simulink model "mppt"  (R2015a)
settings: Solver=ode23tb  StartTime=0.0  StopTime=1.0  RelTol=1e-3
libraries: powerlib x11, simulink x2
settings Model: Creator=Dell  LastModifiedBy=Dell

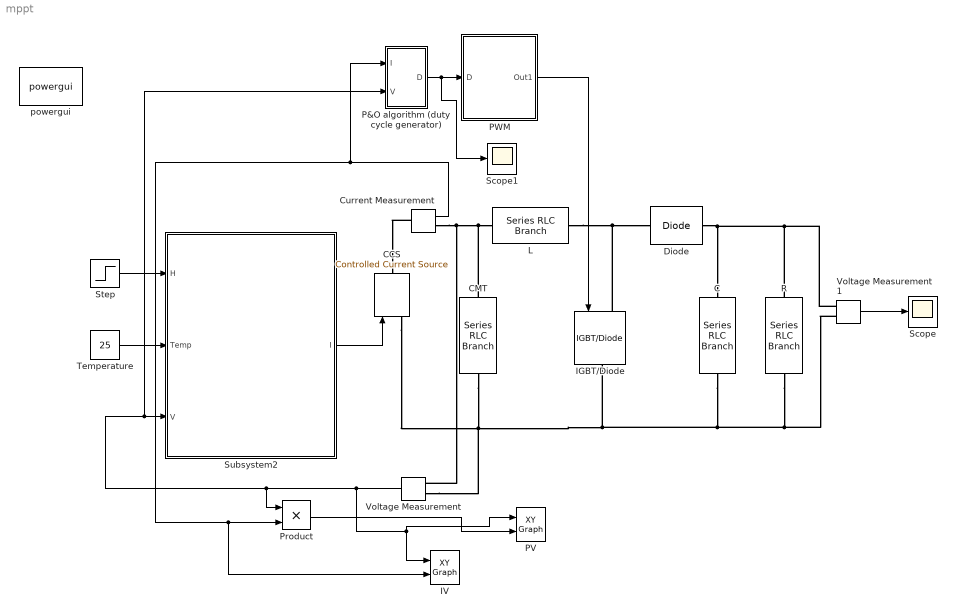
== system mppt ==
  C : powerlib/Elements/Series RLC Branch  LConnTagsString=__new0  RConnTagsString=__new0  BranchType=C  Resistance=1  Inductance=1e-3  SetiL0=off  InitialCurrent=0  Capacitance=1000e-6  Setx0=off  InitialVoltage=0  Measurements=None
  CCS : powerlib/Electrical Sources/Controlled Current Source  Initialize=on  Source_Type=AC  Amplitude=0  Phase=0  Frequency=0  Measurements=None
  CMT : powerlib/Elements/Series RLC Branch  LConnTagsString=__new0  RConnTagsString=__new0  BranchType=C  Resistance=1  Inductance=1e-3  SetiL0=off  InitialCurrent=0  Capacitance=1000e-6  Setx0=off  InitialVoltage=0  Measurements=None
  Current Measurement : powerlib/Measurements/Current Measurement  PhasorSimulation=off  OutputType=Complex  PSBequivalent=0
  Diode : powerlib/Power Electronics/Diode  Ron=0.001  Lon=0  Vf=0.8  IC=0  UseSnubber=off  Rs=500  Cs=250e-9  Measurements=off
  IGBT/Diode : powerlib/Power Electronics/IGBT//Diode  Ron=1e-3  Rs=1e5  Cs=inf  Measurements=off
  IV : simulink/Sinks/XY Graph  xmin=0  xmax=30  ymin=0  ymax=8  st=-1
  L : powerlib/Elements/Series RLC Branch  LConnTagsString=__new0  RConnTagsString=__new0  BranchType=L  Resistance=1  Inductance=4e-4  SetiL0=off  InitialCurrent=0  Capacitance=1e-6  Setx0=off  InitialVoltage=0  Measurements=None
  P&O algorithm (duty cycle generator) : Subsystem
  PV : simulink/Sinks/XY Graph  xmin=0  xmax=20  ymin=0  ymax=75  st=-1
  PWM : Subsystem
  Product : Product
  R : powerlib/Elements/Series RLC Branch  LConnTagsString=__new0  RConnTagsString=__new0  BranchType=R  Resistance=5  Inductance=1e-3  SetiL0=off  InitialCurrent=0  Capacitance=1e-6  Setx0=off  InitialVoltage=0  Measurements=None
  Scope : Scope
      settings: YMin=18.2  YMax=20.2
  Scope1 : Scope
      settings: YMax=-1.75
  Step : Step  Time=0.5  Before=600  After=1000  SampleTime=0
  Subsystem2 : Subsystem
  Temperature : Constant  Value=25
  Voltage Measurement : powerlib/Measurements/Voltage Measurement  PhasorSimulation=off  OutputType=Complex  PSBequivalent=0
  Voltage Measurement1 : powerlib/Measurements/Voltage Measurement  PhasorSimulation=off  OutputType=Complex  PSBequivalent=0
  powergui : powerlib/powergui  Priority=1  SimulationMode=Continuous  SolverType=Tustin/Backward Euler (TBE)  SampleTime=50e-6  frequency=60  SPID=off  DisableSnubberDevices=off  DisableRonSwitches=off  DisableVfSwitches=off  SwTol=0  DisplayEquations=off  Interpol=off  methode=off  Ts=100  FunctionMessages=off  echomessages=off  HookPort=off  EnableUseOfTLC=off  x0status=blocks  frequencyindice=0  Pbase=100e6  ErrMax=1e-4  Iterations=50  UnitsV=kV  UnitsW=MW  buscounter=0  RestoreLinks=warning  ResistiveCurrentMeasurement=off  Frange=[0:2:500]  Ylog=off  Xlog=on  ShowGrid=off  save=off  variable=ZData  structure=0  ZoomFFT=off  StartTime=0.0  cycles=1  DisplayStyle=1  fundamental=60  FreqAxis=off  MaxFrequency=1000  frequencyindicesteady=1  RmsSteady=1  display=off
  wires:
  Subsystem2/1(I) -> CCS/1
  Voltage Measurement/1 -> IV/1, PV/1, Product/1, P&O algorithm (duty cycle generator)/2(V), Subsystem2/3(V)
  Voltage Measurement1/1 -> Scope/1
  Step/1 -> Subsystem2/1(H)
  Temperature/1 -> Subsystem2/2(Temp)
  Current Measurement/1 -> IV/2, Product/2, P&O algorithm (duty cycle generator)/1(I)
  P&O algorithm (duty cycle generator)/1(D) -> Scope1/1, PWM/1(D)
  PWM/1(Out1) -> IGBT/Diode/1
  Product/1 -> PV/2
  connections:
  L/LConn1 -- Current Measurement/RConn1 -- Voltage Measurement/LConn1 -- CMT/LConn1
  L/RConn1 -- IGBT/Diode/LConn1 -- Diode/LConn1
  CCS/LConn1 -- Voltage Measurement/LConn2 -- CMT/RConn1 -- R/RConn1 -- Voltage Measurement1/LConn2 -- C/RConn1 -- IGBT/Diode/RConn1
  Diode/RConn1 -- R/LConn1 -- Voltage Measurement1/LConn1 -- C/LConn1
  Current Measurement/LConn1 -- CCS/RConn1

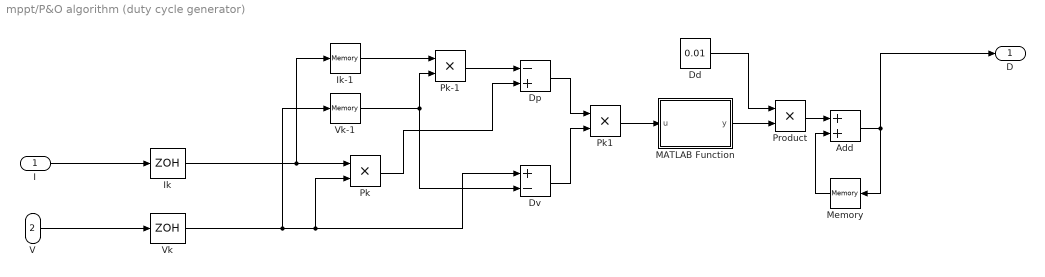
== system mppt/P&O algorithm (duty cycle generator) ==
  I : Inport
  V : Inport  Port=2
  Add : Sum
  Dd : Constant  Value=0.01
  Dp : Sum  Inputs=-+
  Dv : Sum  Inputs=+-
  Ik : ZeroOrderHold  SampleTime=0.001
  Ik-1 : Memory
  MATLAB Function : MATLAB Function  TreatAsAtomicUnit=on
  Memory : Memory
  Pk : Product
  Pk-1 : Product
  Pk1 : Product
  Product : Product
  Vk : ZeroOrderHold  SampleTime=0.001
  Vk-1 : Memory
  D : Outport
  wires:
  Product/1 -> Add/1
  V/1 -> Vk/1
  Add/1 -> D/1, Memory/1
  Memory/1 -> Add/2
  Pk1/1 -> MATLAB Function/1(u)
  Ik/1 -> Pk/1, Ik-1/1
  Dv/1 -> Pk1/2
  Vk/1 -> Dv/1, Pk/2, Vk-1/1
  I/1 -> Ik/1
  Pk/1 -> Dp/2
  Dp/1 -> Pk1/1
  Pk-1/1 -> Dp/1
  MATLAB Function/1(y) -> Product/2
  Ik-1/1 -> Pk-1/1
  Vk-1/1 -> Dv/2, Pk-1/2
  Dd/1 -> Product/1

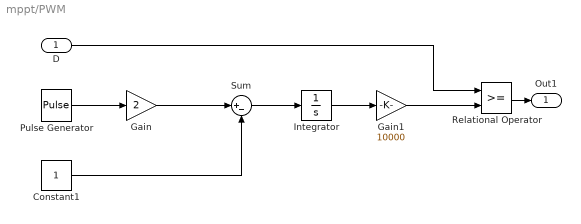
== system mppt/PWM ==
  D : Inport
  Constant1 : Constant
  Gain : Gain  Gain=2
  Gain1 : Gain  Gain=10000
  Integrator : Integrator
  Pulse Generator : DiscretePulseGenerator  PulseType=Time based  Period=0.0002  PulseWidth=50
  Relational Operator : RelationalOperator  OutDataTypeStr=boolean
  Sum : Sum  Inputs=|+-
  Out1 : Outport
  wires:
  Gain1/1 -> Relational Operator/2
  Constant1/1 -> Sum/2
  D/1 -> Relational Operator/1
  Pulse Generator/1 -> Gain/1
  Relational Operator/1 -> Out1/1
  Integrator/1 -> Gain1/1
  Sum/1 -> Integrator/1
  Gain/1 -> Sum/1

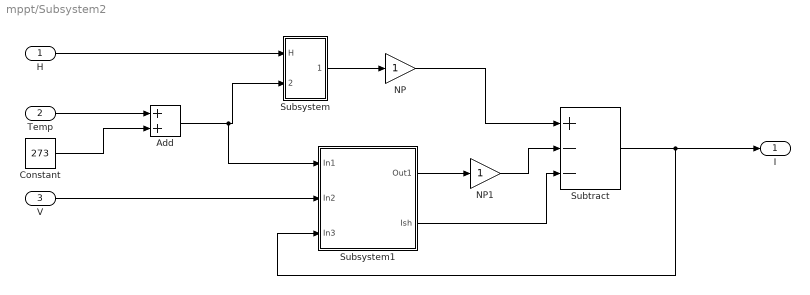
== system mppt/Subsystem2 ==
  H : Inport
  Temp : Inport  Port=2
  V : Inport  Port=3
  Add : Sum
  Constant : Constant  Value=273
  NP : Gain
  NP1 : Gain
  Subsystem : Subsystem
  Subsystem1 : Subsystem
  Subtract : Sum  Inputs=+--
  I : Outport
  wires:
  Subsystem1/1(Out1) -> NP1/1
  Subsystem1/2(Ish) -> Subtract/3
  NP/1 -> Subtract/1
  Subsystem/1(Igh) -> NP/1
  NP1/1 -> Subtract/2
  V/1 -> Subsystem1/2(In2)
  Subtract/1 -> I/1, Subsystem1/3(In3)
  H/1 -> Subsystem/1(H)
  Temp/1 -> Add/1
  Add/1 -> Subsystem1/1(In1), Subsystem/2(Temp)
  Constant/1 -> Add/2

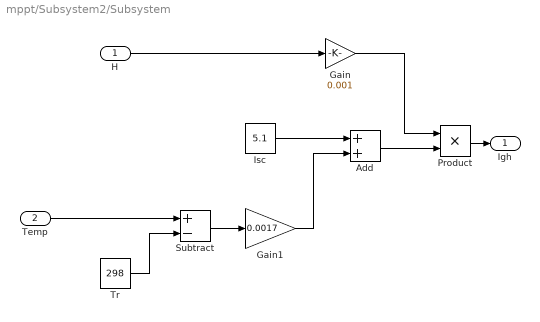
== system mppt/Subsystem2/Subsystem ==
  H : Inport
  Temp : Inport  Port=2
  Add : Sum
  Gain : Gain  Gain=0.001
  Gain1 : Gain  Gain=0.0017
  Isc : Constant  Value=5.1
  Product : Product
  Subtract : Sum  Inputs=+-
  Tr : Constant  Value=298
  Igh : Outport
  wires:
  Add/1 -> Product/2
  Tr/1 -> Subtract/2
  Isc/1 -> Add/1
  H/1 -> Gain/1
  Gain1/1 -> Add/2
  Product/1 -> Igh/1
  Subtract/1 -> Gain1/1
  Temp/1 -> Subtract/1
  Gain/1 -> Product/1

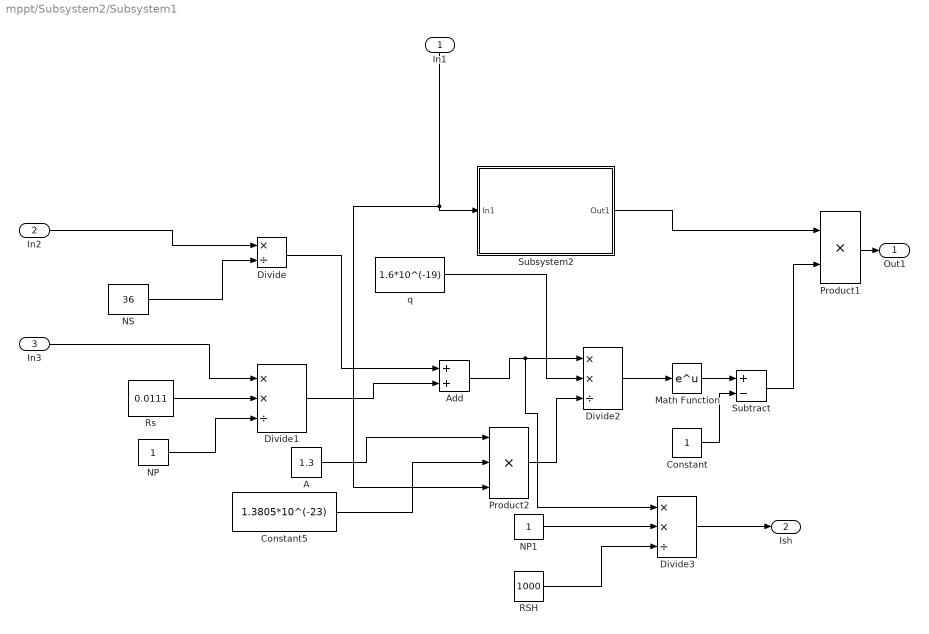
== system mppt/Subsystem2/Subsystem1 ==
  In1 : Inport
  In2 : Inport  Port=2
  In3 : Inport  Port=3
  A : Constant  Value=1.3
  Add : Sum
  Constant : Constant
  Constant5 : Constant  Value=1.3805*10^(-23)
  Divide : Product  Inputs=*/
  Divide1 : Product  Inputs=**/
  Divide2 : Product  Inputs=**/
  Divide3 : Product  Inputs=**/
  Math Function : Math  SaturateOnIntegerOverflow=on
  NP : Constant
  NP1 : Constant
  NS : Constant  Value=36
  Product1 : Product
  Product2 : Product  Inputs=3
  RSH : Constant  Value=1000
  Rs : Constant  Value=0.0111
  Subsystem2 : Subsystem
  Subtract : Sum  Inputs=+-
  q : Constant  Value=1.6*10^(-19)
  Out1 : Outport
  Ish : Outport  Port=2
  wires:
  Rs/1 -> Divide1/2
  In3/1 -> Divide1/1
  Subtract/1 -> Product1/2
  Divide1/1 -> Add/2
  NS/1 -> Divide/2
  Divide2/1 -> Math Function/1
  Add/1 -> Divide3/1, Divide2/1
  NP/1 -> Divide1/3
  In2/1 -> Divide/1
  A/1 -> Product2/1
  Constant5/1 -> Product2/2
  Product1/1 -> Out1/1
  In1/1 -> Product2/3, Subsystem2/1(In1)
  Product2/1 -> Divide2/3
  q/1 -> Divide2/2
  Math Function/1 -> Subtract/1
  Subsystem2/1(Out1) -> Product1/1
  Constant/1 -> Subtract/2
  Divide/1 -> Add/1
  NP1/1 -> Divide3/2
  RSH/1 -> Divide3/3
  Divide3/1 -> Ish/1

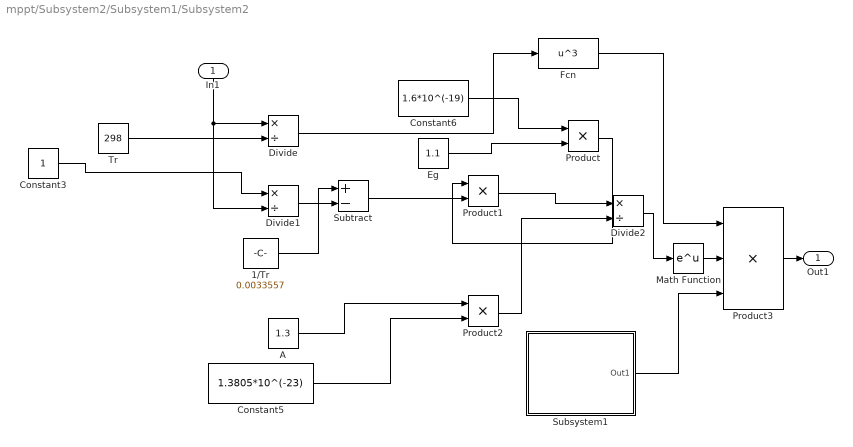
== system mppt/Subsystem2/Subsystem1/Subsystem2 ==
  In1 : Inport
  1/Tr : Constant  Value=0.0033557
  A : Constant  Value=1.3
  Constant3 : Constant
  Constant5 : Constant  Value=1.3805*10^(-23)
  Constant6 : Constant  Value=1.6*10^(-19)
  Divide : Product  Inputs=*/
  Divide1 : Product  Inputs=*/
  Divide2 : Product  Inputs=*/
  Eg : Constant  Value=1.1
  Fcn : Fcn  Expr=u^3
  Math Function : Math  SaturateOnIntegerOverflow=on
  Product : Product
  Product1 : Product
  Product2 : Product
  Product3 : Product  Inputs=3
  Subsystem1 : Subsystem
  Subtract : Sum  Inputs=+-
  Tr : Constant  Value=298
  Out1 : Outport
  wires:
  Subtract/1 -> Product1/2
  Constant6/1 -> Product/1
  Product1/1 -> Divide2/1
  Constant5/1 -> Product2/2
  Fcn/1 -> Product3/1
  Constant3/1 -> Divide1/1
  A/1 -> Product2/1
  Product2/1 -> Divide2/2
  Eg/1 -> Product/2
  Product/1 -> Product1/1
  1/Tr/1 -> Subtract/1
  Divide1/1 -> Subtract/2
  Divide/1 -> Fcn/1
  Product3/1 -> Out1/1
  In1/1 -> Divide/1, Divide1/2
  Tr/1 -> Divide/2
  Subsystem1/1(Out1) -> Product3/3
  Divide2/1 -> Math Function/1
  Math Function/1 -> Product3/2

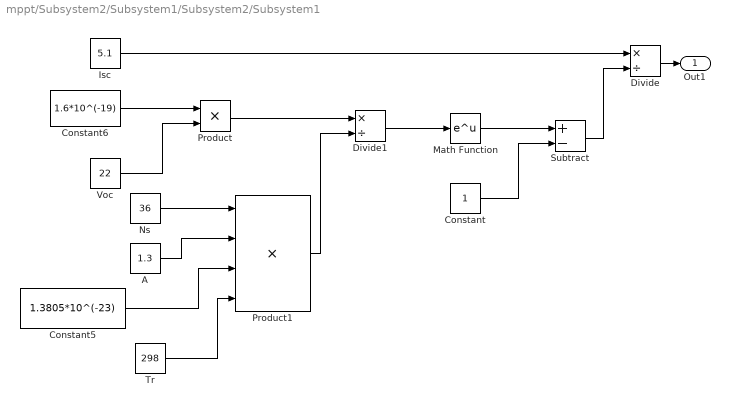
== system mppt/Subsystem2/Subsystem1/Subsystem2/Subsystem1 ==
  A : Constant  Value=1.3
  Constant : Constant
  Constant5 : Constant  Value=1.3805*10^(-23)
  Constant6 : Constant  Value=1.6*10^(-19)
  Divide : Product  Inputs=*/
  Divide1 : Product  Inputs=*/
  Isc : Constant  Value=5.1
  Math Function : Math  SaturateOnIntegerOverflow=on
  Ns : Constant  Value=36
  Product : Product
  Product1 : Product  Inputs=4
  Subtract : Sum  Inputs=+-
  Tr : Constant  Value=298
  Voc : Constant  Value=22
  Out1 : Outport
  wires:
  Math Function/1 -> Subtract/1
  Constant/1 -> Subtract/2
  Subtract/1 -> Divide/2
  Divide/1 -> Out1/1
  Tr/1 -> Product1/4
  Voc/1 -> Product/2
  Ns/1 -> Product1/1
  Product/1 -> Divide1/1
  Constant6/1 -> Product/1
  Constant5/1 -> Product1/3
  Divide1/1 -> Math Function/1
  A/1 -> Product1/2
  Product1/1 -> Divide1/2
  Isc/1 -> Divide/1

== matlab function mppt/P&O algorithm (duty cycle generator)/MATLAB Function ==
  data: u input; y output
function y = fcn(u)
y=0;
if(u==0)
    y=0;
end
if(u>0)
    y=-1;
end
if(u<0)
    y=1;
end
